simulink model "MeasModelCompare_intake"  (R2014b)
settings: Solver=ode45  StartTime=0.0  StopTime=10.0  RelTol=1e-3
values from neighbouring files (symbols this model uses):
  AirStep =     [AirStep.mat]
  n_0 = x(1)    [Init_Project1.m]
  n_1 = x(2)    [Init_Project1.m]
  n_2 = x(3)    [Init_Project1.m]
  n_cyl = EngineMap.engine.n_cyl    [Init_Project1.m]
  n_r = EngineMap.engine.n_r    [Init_Project1.m]    (also in Project1b.m = 2)
  R_air = EngineMap.airfuel.R_air    [Init_Project1.m]
  T_hat_im = x(1)    [Init_Project1.m]
  V_d = 2*a*pi*B^2/4    [Init_Project1.m]
  V_im = EngineMap.engine.V_im    [Init_Project1.m]
settings Model: Creator=danfa688  LastModifiedBy=danfa688

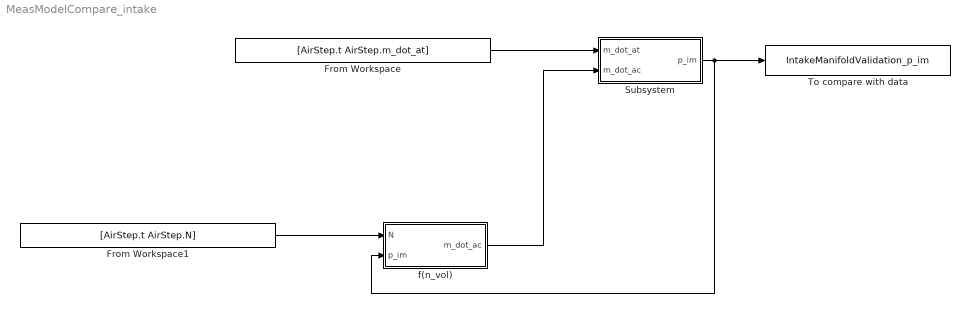
== system MeasModelCompare_intake ==
  From Workspace : FromWorkspace  VariableName=[AirStep.t AirStep.m_dot_at]  SampleTime=0
  From Workspace1 : FromWorkspace  VariableName=[AirStep.t AirStep.N]  SampleTime=0
  Subsystem : Subsystem
  To compare with data : ToWorkspace  VariableName=IntakeManifoldValidation_p_im  SaveFormat=Structure With Time  SampleTime=-1
  f(n_vol) : Subsystem
  wires:
  From Workspace/1 -> Subsystem/1(m_dot_at)
  f(n_vol)/1(m_dot_ac) -> Subsystem/2(m_dot_ac)
  From Workspace1/1 -> f(n_vol)/1(N)
  Subsystem/1(p_im) -> To compare with data/1, f(n_vol)/2(p_im)

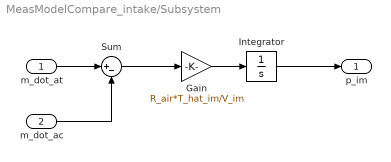
== system MeasModelCompare_intake/Subsystem ==
  m_dot_at : Inport
  m_dot_ac : Inport  Port=2
  Gain : Gain  Gain=R_air*T_hat_im/V_im
  Integrator : Integrator  InitialCondition=AirStep.p_im(1)
  Sum : Sum  Inputs=|+-
  p_im : Outport
  wires:
  m_dot_ac/1 -> Sum/2
  m_dot_at/1 -> Sum/1
  Sum/1 -> Gain/1
  Gain/1 -> Integrator/1
  Integrator/1 -> p_im/1

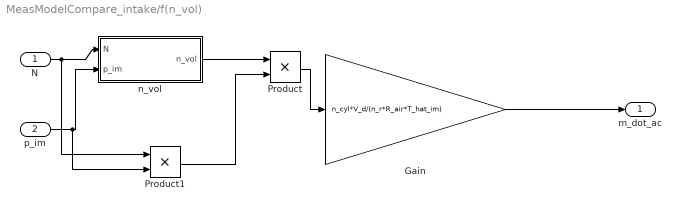
== system MeasModelCompare_intake/f(n_vol) ==
  N : Inport
  p_im : Inport  Port=2
  Gain : Gain  Gain=n_cyl*V_d/(n_r*R_air*T_hat_im)
  Product : Product
  Product1 : Product
  n_vol : Subsystem
  m_dot_ac : Outport
  wires:
  N/1 -> Product1/1, n_vol/1(N)
  p_im/1 -> Product1/2, n_vol/2(p_im)
  n_vol/1(n_vol) -> Product/1
  Product1/1 -> Product/2
  Product/1 -> Gain/1
  Gain/1 -> m_dot_ac/1

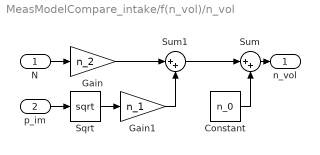
== system MeasModelCompare_intake/f(n_vol)/n_vol ==
  N : Inport
  p_im : Inport  Port=2
  Constant : Constant  Value=n_0
  Gain : Gain  Gain=n_2
  Gain1 : Gain  Gain=n_1
  Sqrt : Sqrt  SaturateOnIntegerOverflow=on
  Sum : Sum  Inputs=|++
  Sum1 : Sum  Inputs=|++
  n_vol : Outport
  wires:
  N/1 -> Gain/1
  p_im/1 -> Sqrt/1
  Constant/1 -> Sum/2
  Sqrt/1 -> Gain1/1
  Sum/1 -> n_vol/1
  Gain/1 -> Sum1/1
  Sum1/1 -> Sum/1
  Gain1/1 -> Sum1/2
